simulink model "Chu_Isfar_Proj1_Part1_v1"  (R2022b)
settings: Solver=VariableStepAuto  StartTime=0.0  StopTime=12  RelTol=1e-9
settings Model: Creator=aspar  LastModifiedBy=aspar
settings DebuggingCC: AlgebraicLoopMsg=none

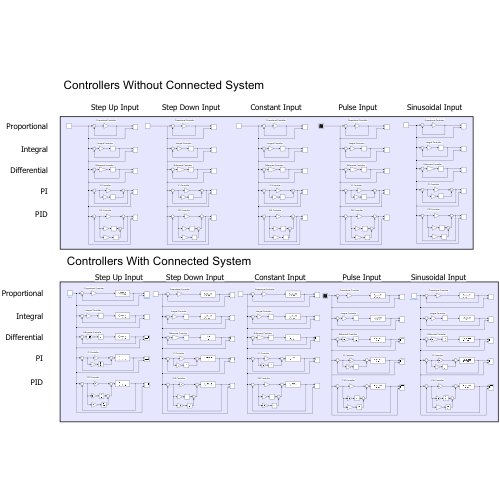
[thumbnail: Simulink's stored preview of the top-level diagram]
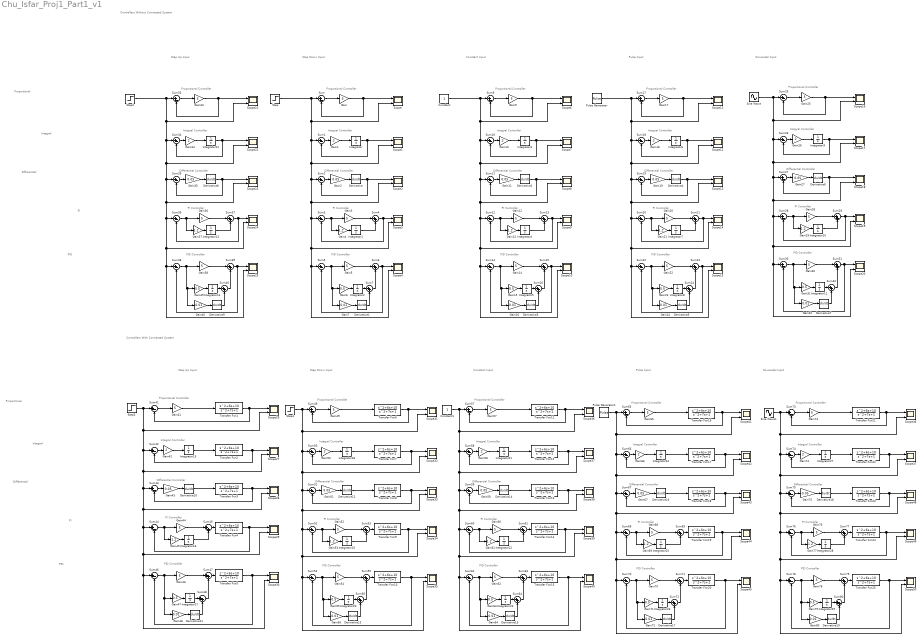
== system Chu_Isfar_Proj1_Part1_v1 ==
  note: Step Up Input
  note: Controllers Without Connected System
  note: PID Controller
  note: PI Controller
  note: Differential Controller
  note: Integral Controller
  note: Proportional Controller
  note: PI Controller
  note: PID Controller
  note: Proportional Controller
  note: Integral Controller
  note: Differential Controller
  note: PI Controller
  note: PID Controller
  note: Proportional Controller
  note: Integral Controller
  note: Differential Controller
  note: PI Controller
  note: PID Controller
  note: Proportional Controller
  note: Integral Controller
  note: Differential Controller
  note: PI Controller
  note: PID Controller
  note: Proportional Controller
  note: Integral Controller
  note: Differential Controller
  note: Integral Controller
  note: Differential Controller
  note: PID Controller
  note: PI Controller
  note: Proportional Controller
  note: Proportional Controller
  note: Integral Controller
  note: PI Controller
  note: Differential Controller
  note: PID Controller
  note: Proportional Controller
  note: Integral Controller
  note: PI Controller
  note: Differential Controller
  note: PID Controller
  note: Step Down Input
  note: Constant Input
  note: Pulse Input
  note: Sinusoidal Input
  note: Differential Controller
  note: Integral Controller
  note: PI Controller
  note: Proportional Controller
  note: PID Controller
  note: Integral Controller
  note: Differential Controller
  note: Proportional Controller
  note: PID Controller
  note: PI Controller
  note: Controllers With Connected System
  note: Proportional
  note: Integral
  note: Differential
  note: PI
  note: PID
  note: Integral
  note: Proportional
  note: PI
  note: Differential
  note: PID
  note: Constant Input
  note: Step Down Input
  note: Pulse Input
  note: Sinusoidal Input
  note: Step Up Input
  Constant : Constant
  Constant1 : Constant
  Derivative{,1..19} (20 alike) : Derivative
  Gain{,3,5,9,12,14,17,20,22,25,28,30,33,36,38,41,44,46,49,52,54,57,60,62,65,68,70,73,76,78} (30 alike) : Gain  Gain=5
  Gain{1,10,18,26,34,42,50,58,66,74} (10 alike) : Gain  Gain=2
  Gain{2,11,19,27,35,43,51,59,67,75} (10 alike) : Gain  Gain=0.05
  Gain{4,13,21,29,37,45,53,61,69,77} (10 alike) : Gain  Gain=1.2
  Gain{6,15,23,31,39,47,55,63,71,79} (10 alike) : Gain  Gain=0.5
  Gain{7,16,24,32,40,48,56,64,72,80} (10 alike) : Gain  Gain=0.01
  Integrator{,1..29} (30 alike) : Integrator
  Pulse Generator : DiscretePulseGenerator  PulseType=Time based  Period=10  PulseWidth=50
  Pulse Generator1 : DiscretePulseGenerator  PulseType=Time based  Period=10  PulseWidth=50
  Scope{,1..4,6..50} (50 alike) : Scope  NumInputPorts=2
  Sine Wave : Sin  SampleTime=0
  Sine Wave1 : Sin  SampleTime=0
  Step : Step  Time=5  Before=1  After=0  SampleTime=0
  Step2 : Step  Time=5  SampleTime=0
  Step3 : Step  Time=5  SampleTime=0
  Step4 : Step  Time=5  Before=1  After=0  SampleTime=0
  Sum{,1..3,5,9..12,14,17..20,22,25..28,30,33..36,38,41..44,46,49..52,54,57..60,62,65..68,70,73..76,78} (50 alike) : Sum  Inputs=|+-
  Sum{4,6..7,13,15..16,21,23..24,29,31..32,37,39..40,45,47..48,53,55..56,61,63..64,69,71..72,77,79..80} (30 alike) : Sum  Inputs=|++
  Transfer Fcn{1..25} (25 alike) : TransferFcn  Numerator=[1 6 10]  Denominator=[1 7 1]
  wires:
  Sum/1 -> Gain/1
  Gain/1 -> Scope/1, Sum/2
  Sum1/1 -> Gain1/1
  Gain1/1 -> Integrator/1
  Integrator/1 -> Scope1/1, Sum1/2
  Derivative/1 -> Scope2/1, Sum2/2
  Gain2/1 -> Derivative/1
  Sum2/1 -> Gain2/1
  Sum3/1 -> Gain4/1, Gain3/1
  Gain4/1 -> Integrator1/1
  Integrator1/1 -> Sum4/2
  Sum4/1 -> Sum3/2, Scope3/1
  Gain3/1 -> Sum4/1
  Sum6/1 -> Scope4/1, Sum5/2
  Gain5/1 -> Sum6/1
  Gain6/1 -> Integrator2/1
  Sum7/1 -> Sum6/2
  Integrator2/1 -> Sum7/1
  Gain7/1 -> Derivative1/1
  Sum5/1 -> Gain7/1, Gain6/1, Gain5/1
  Derivative1/1 -> Sum7/2
  Step/1 -> Scope4/2, Sum5/1, Scope3/2, Sum3/1, Scope2/2, Sum2/1, Scope1/2, Sum1/1, Scope/2, Sum/1
  Sum13/1 -> Sum12/2, Scope9/1
  Gain12/1 -> Sum13/1
  Derivative2/1 -> Scope8/1, Sum11/2
  Integrator5/1 -> Sum16/1
  Integrator4/1 -> Sum13/2
  Sum9/1 -> Gain9/1
  Gain11/1 -> Derivative2/1
  Gain13/1 -> Integrator4/1
  Integrator3/1 -> Scope7/1, Sum10/2
  Sum16/1 -> Sum15/2
  Derivative3/1 -> Sum16/2
  Gain15/1 -> Integrator5/1
  Sum14/1 -> Gain16/1, Gain15/1, Gain14/1
  Gain9/1 -> Scope6/1, Sum9/2
  Gain14/1 -> Sum15/1
  Sum15/1 -> Scope10/1, Sum14/2
  Sum11/1 -> Gain11/1
  Gain10/1 -> Integrator3/1
  Gain16/1 -> Derivative3/1
  Sum10/1 -> Gain10/1
  Sum12/1 -> Gain13/1, Gain12/1
  Constant/1 -> Scope10/2, Sum14/1, Scope9/2, Sum12/1, Scope8/2, Sum11/1, Scope7/2, Sum10/1, Scope6/2, Sum9/1
  Sum21/1 -> Sum20/2, Scope14/1
  Gain20/1 -> Sum21/1
  Derivative4/1 -> Scope13/1, Sum19/2
  Integrator8/1 -> Sum24/1
  Integrator7/1 -> Sum21/2
  Sum17/1 -> Gain17/1
  Gain19/1 -> Derivative4/1
  Gain21/1 -> Integrator7/1
  Integrator6/1 -> Scope12/1, Sum18/2
  Sum24/1 -> Sum23/2
  Derivative5/1 -> Sum24/2
  Gain23/1 -> Integrator8/1
  Sum22/1 -> Gain24/1, Gain23/1, Gain22/1
  Gain17/1 -> Scope11/1, Sum17/2
  Gain22/1 -> Sum23/1
  Sum23/1 -> Scope15/1, Sum22/2
  Sum19/1 -> Gain19/1
  Gain18/1 -> Integrator6/1
  Gain24/1 -> Derivative5/1
  Sum18/1 -> Gain18/1
  Sum20/1 -> Gain21/1, Gain20/1
  Pulse Generator/1 -> Scope15/2, Sum22/1, Scope14/2, Sum20/1, Scope13/2, Sum19/1, Scope12/2, Sum18/1, Scope11/2, Sum17/1
  Sum29/1 -> Sum28/2, Scope19/1
  Gain28/1 -> Sum29/1
  Derivative6/1 -> Scope18/1, Sum27/2
  Integrator11/1 -> Sum32/1
  Integrator10/1 -> Sum29/2
  Sum25/1 -> Gain25/1
  Gain27/1 -> Derivative6/1
  Gain29/1 -> Integrator10/1
  Integrator9/1 -> Scope17/1, Sum26/2
  Sum32/1 -> Sum31/2
  Derivative7/1 -> Sum32/2
  Gain31/1 -> Integrator11/1
  Sum30/1 -> Gain32/1, Gain31/1, Gain30/1
  Gain25/1 -> Scope16/1, Sum25/2
  Gain30/1 -> Sum31/1
  Sum31/1 -> Scope20/1, Sum30/2
  Sum27/1 -> Gain27/1
  Gain26/1 -> Integrator9/1
  Gain32/1 -> Derivative7/1
  Sum26/1 -> Gain26/1
  Sum28/1 -> Gain29/1, Gain28/1
  Sine Wave/1 -> Scope20/2, Sum30/1, Scope19/2, Sum28/1, Scope18/2, Sum27/1, Scope17/2, Sum26/1, Scope16/2, Sum25/1
  Sum37/1 -> Sum36/2, Scope24/1
  Gain36/1 -> Sum37/1
  Derivative8/1 -> Scope23/1, Sum35/2
  Integrator14/1 -> Sum40/1
  Integrator13/1 -> Sum37/2
  Sum33/1 -> Gain33/1
  Gain35/1 -> Derivative8/1
  Gain37/1 -> Integrator13/1
  Integrator12/1 -> Scope22/1, Sum34/2
  Sum40/1 -> Sum39/2
  Derivative9/1 -> Sum40/2
  Gain39/1 -> Integrator14/1
  Sum38/1 -> Gain40/1, Gain39/1, Gain38/1
  Gain33/1 -> Scope21/1, Sum33/2
  Gain38/1 -> Sum39/1
  Sum39/1 -> Scope25/1, Sum38/2
  Sum35/1 -> Gain35/1
  Gain34/1 -> Integrator12/1
  Gain40/1 -> Derivative9/1
  Sum34/1 -> Gain34/1
  Sum36/1 -> Gain37/1, Gain36/1
  Step2/1 -> Scope25/2, Sum38/1, Scope24/2, Sum36/1, Scope23/2, Sum35/1, Scope22/2, Sum34/1, Scope21/2, Sum33/1
  Sum42/1 -> Gain42/1
  Step3/1 -> Sum46/1, Scope30/2, Scope29/2, Sum44/1, Scope28/2, Sum43/1, Scope27/2, Sum42/1, Scope26/2, Sum41/1
  Gain43/1 -> Derivative10/1
  Integrator16/1 -> Sum45/2
  Derivative10/1 -> Transfer Fcn3/1
  Sum41/1 -> Gain41/1
  Sum44/1 -> Gain45/1, Gain44/1
  Sum45/1 -> Transfer Fcn4/1
  Integrator17/1 -> Sum48/1
  Gain42/1 -> Integrator15/1
  Sum48/1 -> Sum47/2
  Integrator15/1 -> Transfer Fcn2/1
  Derivative11/1 -> Sum48/2
  Gain45/1 -> Integrator16/1
  Gain48/1 -> Derivative11/1
  Sum46/1 -> Gain48/1, Gain47/1, Gain46/1
  Sum47/1 -> Transfer Fcn5/1
  Gain46/1 -> Sum47/1
  Gain44/1 -> Sum45/1
  Gain41/1 -> Transfer Fcn1/1
  Sum43/1 -> Gain43/1
  Gain47/1 -> Integrator17/1
  Transfer Fcn5/1 -> Sum46/2, Scope30/1
  Transfer Fcn4/1 -> Scope29/1, Sum44/2
  Transfer Fcn3/1 -> Scope28/1, Sum43/2
  Transfer Fcn2/1 -> Scope27/1, Sum42/2
  Transfer Fcn1/1 -> Scope26/1, Sum41/2
  Sum55/1 -> Transfer Fcn10/1
  Sum51/1 -> Gain51/1
  Gain54/1 -> Sum55/1
  Gain52/1 -> Sum53/1
  Sum54/1 -> Gain56/1, Gain55/1, Gain54/1
  Derivative13/1 -> Sum56/2
  Sum52/1 -> Gain53/1, Gain52/1
  Gain49/1 -> Transfer Fcn6/1
  Sum53/1 -> Transfer Fcn9/1
  Integrator20/1 -> Sum56/1
  Integrator18/1 -> Transfer Fcn7/1
  Integrator19/1 -> Sum53/2
  Gain51/1 -> Derivative12/1
  Gain55/1 -> Integrator20/1
  Step4/1 -> Sum54/1, Scope35/2, Scope34/2, Sum52/1, Scope33/2, Sum51/1, Scope32/2, Sum50/1, Scope31/2, Sum49/1
  Sum49/1 -> Gain49/1
  Gain50/1 -> Integrator18/1
  Sum50/1 -> Gain50/1
  Gain56/1 -> Derivative13/1
  Transfer Fcn7/1 -> Scope32/1, Sum50/2
  Transfer Fcn10/1 -> Sum54/2, Scope35/1
  Sum56/1 -> Sum55/2
  Gain53/1 -> Integrator19/1
  Transfer Fcn8/1 -> Scope33/1, Sum51/2
  Derivative12/1 -> Transfer Fcn8/1
  Transfer Fcn6/1 -> Scope31/1, Sum49/2
  Transfer Fcn9/1 -> Scope34/1, Sum52/2
  Sum63/1 -> Transfer Fcn15/1
  Sum59/1 -> Gain59/1
  Gain62/1 -> Sum63/1
  Gain60/1 -> Sum61/1
  Sum62/1 -> Gain64/1, Gain63/1, Gain62/1
  Derivative15/1 -> Sum64/2
  Sum60/1 -> Gain61/1, Gain60/1
  Gain57/1 -> Transfer Fcn11/1
  Sum61/1 -> Transfer Fcn14/1
  Integrator23/1 -> Sum64/1
  Integrator21/1 -> Transfer Fcn12/1
  Integrator22/1 -> Sum61/2
  Gain59/1 -> Derivative14/1
  Gain63/1 -> Integrator23/1
  Constant1/1 -> Sum62/1, Scope40/2, Scope39/2, Sum60/1, Scope38/2, Sum59/1, Scope37/2, Sum58/1, Scope36/2, Sum57/1
  Sum57/1 -> Gain57/1
  Gain58/1 -> Integrator21/1
  Sum58/1 -> Gain58/1
  Gain64/1 -> Derivative15/1
  Transfer Fcn12/1 -> Scope37/1, Sum58/2
  Transfer Fcn15/1 -> Sum62/2, Scope40/1
  Sum64/1 -> Sum63/2
  Gain61/1 -> Integrator22/1
  Transfer Fcn13/1 -> Scope38/1, Sum59/2
  Derivative14/1 -> Transfer Fcn13/1
  Transfer Fcn11/1 -> Scope36/1, Sum57/2
  Transfer Fcn14/1 -> Scope39/1, Sum60/2
  Transfer Fcn19/1 -> Scope44/1, Sum68/2
  Gain69/1 -> Integrator25/1
  Transfer Fcn18/1 -> Scope43/1, Sum67/2
  Gain66/1 -> Integrator24/1
  Sum65/1 -> Gain65/1
  Sum66/1 -> Gain66/1
  Integrator25/1 -> Sum69/2
  Gain65/1 -> Transfer Fcn16/1
  Gain71/1 -> Integrator26/1
  Gain67/1 -> Derivative16/1
  Integrator24/1 -> Transfer Fcn17/1
  Integrator26/1 -> Sum72/1
  Gain70/1 -> Sum71/1
  Sum68/1 -> Gain69/1, Gain68/1
  Transfer Fcn17/1 -> Scope42/1, Sum66/2
  Transfer Fcn16/1 -> Scope41/1, Sum65/2
  Sum67/1 -> Gain67/1
  Sum69/1 -> Transfer Fcn19/1
  Transfer Fcn20/1 -> Sum70/2, Scope45/1
  Derivative17/1 -> Sum72/2
  Gain72/1 -> Derivative17/1
  Sum72/1 -> Sum71/2
  Gain68/1 -> Sum69/1
  Sum70/1 -> Gain72/1, Gain71/1, Gain70/1
  Sum71/1 -> Transfer Fcn20/1
  Derivative16/1 -> Transfer Fcn18/1
  Pulse Generator1/1 -> Sum70/1, Scope45/2, Scope44/2, Sum68/1, Scope43/2, Sum67/1, Scope42/2, Sum66/1, Scope41/2, Sum65/1
  Derivative18/1 -> Transfer Fcn23/1
  Transfer Fcn25/1 -> Sum78/2, Scope50/1
  Sum77/1 -> Transfer Fcn24/1
  Derivative19/1 -> Sum80/2
  Sum78/1 -> Gain80/1, Gain79/1, Gain78/1
  Sum80/1 -> Sum79/2
  Sum75/1 -> Gain75/1
  Integrator29/1 -> Sum80/1
  Gain75/1 -> Derivative18/1
  Sum76/1 -> Gain77/1, Gain76/1
  Integrator27/1 -> Transfer Fcn22/1
  Transfer Fcn22/1 -> Scope47/1, Sum74/2
  Gain76/1 -> Sum77/1
  Gain79/1 -> Integrator29/1
  Gain73/1 -> Transfer Fcn21/1
  Transfer Fcn21/1 -> Scope46/1, Sum73/2
  Integrator28/1 -> Sum77/2
  Gain74/1 -> Integrator27/1
  Gain78/1 -> Sum79/1
  Gain77/1 -> Integrator28/1
  Sum79/1 -> Transfer Fcn25/1
  Sum74/1 -> Gain74/1
  Gain80/1 -> Derivative19/1
  Transfer Fcn24/1 -> Scope49/1, Sum76/2
  Sum73/1 -> Gain73/1
  Transfer Fcn23/1 -> Scope48/1, Sum75/2
  Sine Wave1/1 -> Sum78/1, Scope50/2, Scope49/2, Sum76/1, Scope48/2, Sum75/1, Scope47/2, Sum74/1, Scope46/2, Sum73/1
